simulink model "MPC"  (R2017a)
settings: Solver=ode3  StartTime=0.0  StopTime=inf  MaxStep=1e-4  RelTol=1e-3
values from neighbouring files (symbols this model uses):
  I1 = 1.17    [sistemacontrolado.m]    (also in sistemacontrolado.mat)
  I2 = 3    [sistemacontrolado.m]    (also in sistemacontrolado.mat)
  R = Ra1    (= 28.8)    [sistemacontrolado.m]    (also in sistemacontrolado.mat)
libraries: powerlib x9, instrumentlib x6, simulink_extras x1, mpclib x1, powerlib_meascontrol x1
settings Model: Creator=MarioAndres  LastModifiedBy=AndrewB
settings DebuggingCC: UnconnectedLineMsg=none
settings RTWCC: GenCodeOnly=on

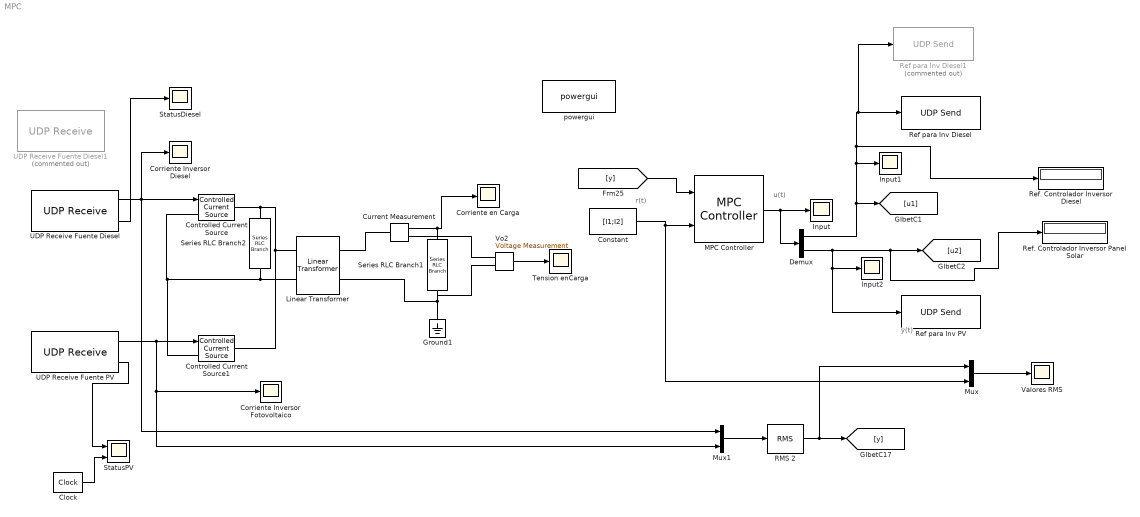
== system MPC ==
  note: u(t)
  note: y(t)
  note: r(t)
  Clock : simulink_extras/Flip Flops/Clock  period=1/60/10000
  Constant : Constant  Value=[I1;I2]
  Controlled Current Source : powerlib/Electrical Sources/Controlled Current Source  Initialize=on  Source_Type=AC  Amplitude=0  Phase=0  Frequency=0  Measurements=None
  Controlled Current Source1 : powerlib/Electrical Sources/Controlled Current Source  Initialize=on  Source_Type=AC  Amplitude=0  Phase=0  Frequency=0  Measurements=None
  Corriente Inversor Diesel : Scope
  Corriente Inversor Fotovoltaico : Scope
  Corriente en Carga : Scope
  Current Measurement : powerlib/Measurements/Current Measurement  PhasorSimulation=off  OutputType=Complex  PSBequivalent=0
  Demux : Demux  Outputs=2
  Ground1 : powerlib/Elements/Ground  LConnTagsString=a
  Input : Scope
  Input1 : Scope
  Input2 : Scope
  Linear Transformer : powerlib/Elements/Linear Transformer  UNITS=SI  NominalPower=[ 1500 60 ]  winding1=[141.2 0 0.01]  winding2=[120 0.004 0.084225]  ThreeWindings=off  winding3=[3.15e+05 0.7938 0.084225]  RmLm=[1.0805e+06 2866]  Measurements=None  DataType=on
  MPC Controller : mpclib/MPC Controller  mpcobj=mpcobj  x0=[]  is_multiple=0  enable_value=0  return_u0=off  ref_from_ws=off  ref_signal_name=[]  ref_preview=on  md_from_ws=off  md_signal_name=[]  md_preview=on  from_project=off  project_file=MPCtask.mat  md_inport=off  mv_inport=off  cost_outport=off  return_sequence=off  return_qpstatus=off  return_state=off  state_inport=off  lims_inport=off  ywt_inport=off  is_designfromscratch=0  uwt_inport=off  duwt_inport=off  rhoeps_inport=off  uref_inport=off  n_ts=0.1  n_mv=2  n_md=0  n_ud=0  n_mo=2  n_uo=0  BlockDataType=double  SampleTimeInherited=off  switch_inport=off
  Mux : Mux  Inputs=2
  Mux1 : Mux  Inputs=2
  RMS 2 : powerlib_meascontrol/Measurements/RMS  TrueRMS=on  Freq=60  RMSInit=0  Ts=1/60/10000
  Ref para Inv Diesel : instrumentlib/UDP Send  Priority=2  Host=169.254.26.197  Port=51004  LocalPort=51005  EnableBlockingMode=on  ByteOrder=BigEndian
      settings: SourceProductName=Instrument Control Toolbox
  Ref para Inv Diesel1 : instrumentlib/UDP Send  Priority=2  Commented=on  Host=localhost  Port=51004  LocalPort=51005  EnableBlockingMode=on  ByteOrder=BigEndian
      settings: SourceProductName=Instrument Control Toolbox
  Ref para Inv PV : instrumentlib/UDP Send  Priority=2  Host=169.254.51.223  Port=51000  LocalPort=51001  EnableBlockingMode=on  ByteOrder=BigEndian
      settings: SourceProductName=Instrument Control Toolbox
  Ref. Controlador Inversor Diesel : Display
  Ref. Controlador Inversor Panel Solar : Display
  Series RLC Branch1 : powerlib/Elements/Series RLC Branch  LConnTagsString=__new0  RConnTagsString=__new0  BranchType=R  Resistance=R  Inductance=25e-3  SetiL0=off  InitialCurrent=0  Capacitance=5.30e-3  Setx0=off  InitialVoltage=0  Measurements=None
  Series RLC Branch2 : powerlib/Elements/Series RLC Branch  LConnTagsString=__new0  RConnTagsString=__new0  BranchType=R  Resistance=1e6  Inductance=25e-3  SetiL0=off  InitialCurrent=0  Capacitance=5.30e-3  Setx0=off  InitialVoltage=0  Measurements=None
  StatusDiesel : Scope
  StatusPV : Scope  NumInputPorts=2
  Tension enCarga : Scope
  UDP Receive Fuente Diesel : instrumentlib/UDP Receive  Host=169.254.26.197  Port=51004  LocalPort=51005  DataSize=1  EnableBlockingMode=off  Timeout=100  SampleTime=-1  DataType=double  ByteOrder=BigEndian
      settings: SourceProductName=Instrument Control Toolbox
  UDP Receive Fuente Diesel1 : instrumentlib/UDP Receive  Commented=on  Host=localhost  Port=51004  LocalPort=51005  DataSize=1  EnableBlockingMode=off  Timeout=100  SampleTime=-1  DataType=double  ByteOrder=BigEndian
      settings: SourceProductName=Instrument Control Toolbox
  UDP Receive Fuente PV : instrumentlib/UDP Receive  Host=169.254.51.223  Port=51000  LocalPort=51001  DataSize=1  EnableBlockingMode=off  Timeout=100  SampleTime=-1  DataType=double  ByteOrder=BigEndian
      settings: SourceProductName=Instrument Control Toolbox
  Valores RMS : Scope
  Vo2 : powerlib/Measurements/Voltage Measurement  PhasorSimulation=off  OutputType=Complex  PSBequivalent=0
  powergui : powerlib/powergui  Priority=1  SimulationMode=Discrete  SampleTime=1/60/10000  frequency=60  Iterations=50  frequencyindice=0  Pbase=100e6  ErrMax=1e-4  UnitsV=kV  UnitsW=MW  buscounter=0  FunctionMessages=off  echomessages=off  EnableUseOfTLC=off  CurrentSourceSwitches=off  DisableSnubberDevices=off  DisableRonSwitches=off  DisableVfSwitches=off  DisplayEquations=off  SolverType=Tustin/Backward Euler (TBE)  Interpol=off  ExternalGateDelay=off  methode=off  Ts=100  x0status=blocks  SPID=on  SwTol=0  HookPort=off  RestoreLinks=warning  ResistiveCurrentMeasurement=off  Frange=[0:2:500]  Ylog=off  Xlog=on  ShowGrid=off  save=off  variable=ZData  structure=0  ZoomFFT=off  StartTime=0.0  cycles=1  DisplayStyle=1  fundamental=60  FreqAxis=off  MaxFrequency=1000  frequencyindicesteady=1  RmsSteady=1  display=off
  wires:
  [y] -> MPC Controller/1
  Demux/2 -> Ref para Inv PV/1, Input2/1, Ref. Controlador Inversor Panel Solar/1, [u2]
  Constant/1 -> Mux/2, MPC Controller/2
  Mux/1 -> Valores RMS/1
  MPC Controller/1 -> Demux/1, Input/1
  Demux/1 -> Ref. Controlador Inversor Diesel/1, Ref para Inv Diesel1/1, Ref para Inv Diesel/1, Input1/1, [u1]
  Vo2/1 -> Tension enCarga/1
  Current Measurement/1 -> Corriente en Carga/1
  Mux1/1 -> RMS 2/1
  UDP Receive Fuente PV/1 -> Controlled Current Source1/1, Corriente Inversor Fotovoltaico/1, Mux1/2
  RMS 2/1 -> Mux/1, [y]
  UDP Receive Fuente PV/2 -> StatusPV/1
  Clock/1 -> StatusPV/2
  UDP Receive Fuente Diesel/1 -> Corriente Inversor Diesel/1, Mux1/1, Controlled Current Source/1
  UDP Receive Fuente Diesel/2 -> StatusDiesel/1
  connections:
  Series RLC Branch1/LConn1 -- Vo2/LConn1 -- Current Measurement/RConn1
  Series RLC Branch1/RConn1 -- Ground1/LConn1 -- Linear Transformer/RConn2 -- Vo2/LConn2
  Linear Transformer/RConn1 -- Current Measurement/LConn1
  Controlled Current Source/RConn1 -- Controlled Current Source1/RConn1 -- Linear Transformer/LConn1 -- Series RLC Branch2/LConn1
  Controlled Current Source/LConn1 -- Controlled Current Source1/LConn1 -- Linear Transformer/LConn2 -- Series RLC Branch2/RConn1
